simulink model "ExC_model"  (R2021b)
settings: Solver=VariableStepAuto  StartTime=0.0  StopTime=45  RelTol=1e-3
libraries: simulink x1
settings Model: Creator=westwick  LastModifiedBy=randy
settings SolverCC: AlgebraicLoopSolver=TrustRegion
settings DebuggingCC: SFMachineParentedDataDiag=warning
settings SFSimCC: CustomCodeUndefinedFunction=UseInterfaceOnly

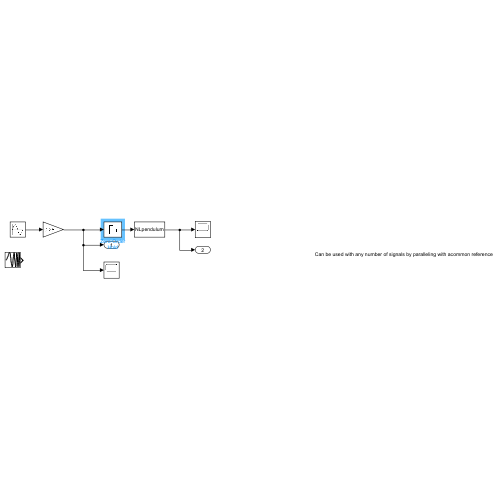
[thumbnail: Simulink's stored preview of the top-level diagram]
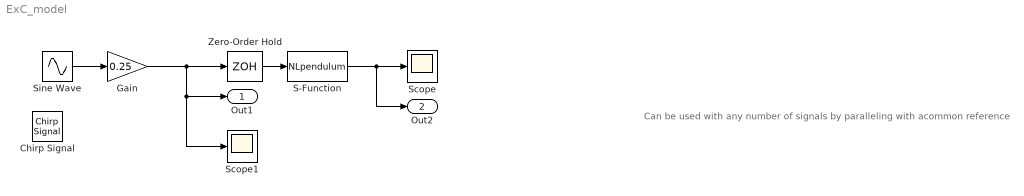
== system ExC_model ==
  note: Can be used with any number of signals by paralleling with acommon reference
  Chirp Signal : simulink/Sources/Chirp Signal  f1=0.2  T=30  f2=2
  Gain : Gain  Gain=0.25
  S-Function : S-Function  FunctionName=NLpendulum  SFunctionDeploymentMode=off  EnableBusSupport=off
  Scope : Scope
  Scope1 : Scope
  Sine Wave : Sin  Frequency=2*pi  SampleTime=0
  Zero-Order Hold : ZeroOrderHold  SampleTime=0.3
  Out1 : Outport  VectorParamsAs1DForOutWhenUnconnected=off
  Out2 : Outport  Port=2  VectorParamsAs1DForOutWhenUnconnected=off
  wires:
  Gain/1 -> Zero-Order Hold/1, Out1/1, Scope1/1
  S-Function/1 -> Out2/1, Scope/1
  Sine Wave/1 -> Gain/1
  Zero-Order Hold/1 -> S-Function/1
